simulink model "machineModel"  (R2021a)
settings: Solver=VariableStepAuto  StartTime=0.0  StopTime=10.0  RelTol=1e-3
settings Model: Creator=ibirl  LastModifiedBy=ibirl

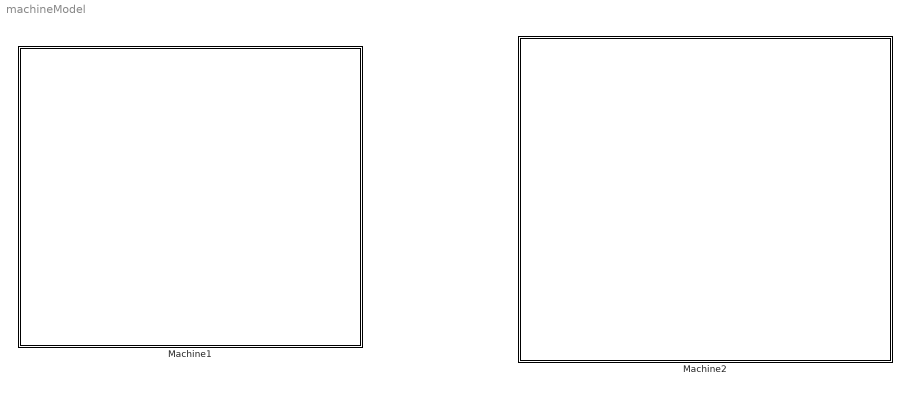
== system machineModel ==
  Machine1 : Stateflow chart  TreatAsAtomicUnit=on
  Machine2 : Stateflow chart  TreatAsAtomicUnit=on

== stateflow chart machineModel/Machine2 ==
  note: If buffer content is zero, we can't leave A until upstream machine has placed a part in the buffer. No part can be drawn from the buffer until then.
  note: This only happens when the first machine fails OR is in a non-productive state (a buffer isn't changing).
  note: The only way to have a zero buffer is if downstream machine removes a part while the upstream hasn't put a part in.
  state A
  note: i.e. upstream is in b, c, ..., g
  note: downstream machine is in A
  note: A represents receiving a part
  note: Have to add logic about getting into and out of this starved/blocked
      | condition
  note: Assumption: infinite space downstream; infinite parts upstream
  state B
  state C
  state D
  note: error trapping code to make sure probabilities of exiting a node add to one.
  note: B,C,D represent processing of part
  note: Model helps us decide expected time to complete a part when good probabilities are chosen
  A -> A [order 2] : [0.413818]{-1}
  D -> A [order 1] : [0.610816]{-1}
  C -> A [order 2] : [0.520216]{-1}
  A -> B [order 1] : [0.586182]{0}
  B -> A [order 1] : [0.778154]{-1}
  C -> D [order 1] : [0.238513]{0}
  B -> C [order 2] : [0.082936]{0}
  B -> B [order 3] : [0.13891]{0}
  C -> C [order 3] : [0.241271]{0}
  D -> D [order 2] : [0.389184]{0}

== stateflow chart machineModel/Machine1 ==
  state a
  state b
  state c
  state d
  state e
  state f
  state g
  a -> a [order 2] : [0.220488]{1}
  g -> a [order 1] : [0.678425]{1}
  f -> a [order 2] : [0.399127]{1}
  e -> a [order 2] : [0.406416]{1}
  a -> b [order 1] : [0.779512]{0}
  b -> a [order 3] : [0.437727]{1}
  c -> a [order 2] : [0.539262]{1}
  d -> a [order 2] : [0.364206]{1}
  f -> g [order 1] : [0.380154]{0}
  e -> f [order 1] : [0.352634]{0}
  b -> c [order 2] : [0.345966]{0}
  c -> d [order 1] : [0.276785]{0}
  d -> e [order 1] : [0.342976]{0}
  b -> b [order 1] : [0.216307]{0}
  c -> c [order 3] : [0.183953]{0}
  d -> d [order 3] : [0.292818]{0}
  e -> e [order 3] : [0.24095]{0}
  f -> f [order 3] : [0.220719]{0}
  g -> g [order 2] : [0.321575]{0}
